simulink subsystem "ExcavatorLidarSensors"  (R2024a)
settings: Solver=VariableStepAuto  StartTime=0.0  StopTime=10.0  RelTol=1e-3
values from neighbouring files (symbols this model uses):
  lidarSampleTime = 0.1    [lidarSensorParameters.mat]
libraries: sim3dphyssensorlib x4
settings Model: Creator=ckammer  LastModifiedBy=ckammer

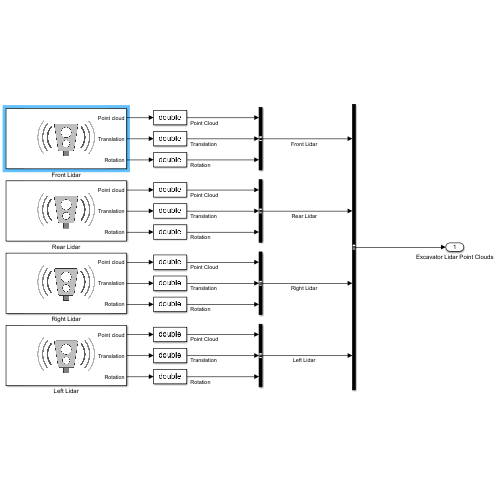
[thumbnail: Simulink's stored preview of the top-level diagram]
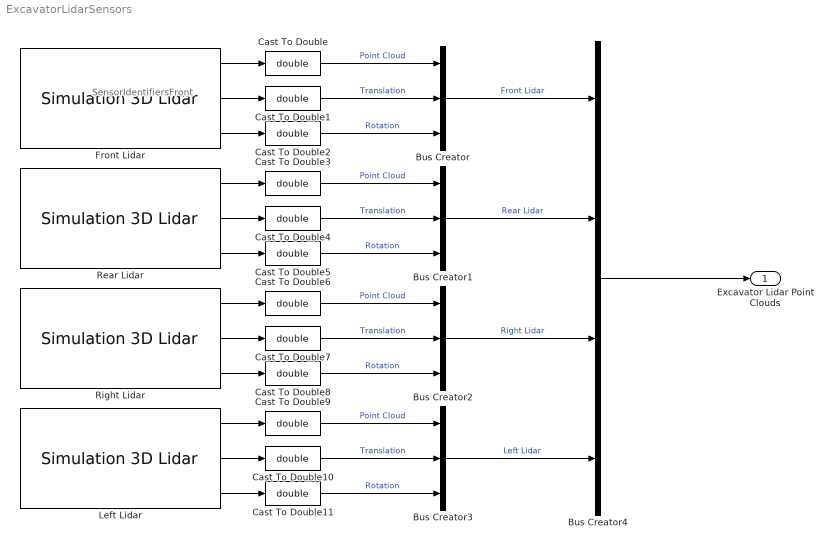
== system ExcavatorLidarSensors ==
  note: SensorIdentifiersFront
  Bus Creator{,1..3} (4 alike) : BusCreator  Inputs=3
  Bus Creator4 : BusCreator  Inputs=4
  Cast To Double{,1..11} (12 alike) : DataTypeConversion  OutDataTypeStr=double  SaturateOnIntegerOverflow=off  RndMeth=Floor
  Front Lidar : sim3dphyssensorlib/Simulation 3D Lidar  Priority=1  sensorTag=Sim3dSensorSensorIdentifiers.LidarSensorFront  sensorId=SensorIdentifiers.LidarSensorFront  sensorName=Sim3dSensorSensorIdentifiers.LidarSensorFront  vehTagList={'Scene Origin'}  vehTag=Scene Origin  mountLoc=Origin  offsetFlag=on  tmountOffset=lidarSensorOffsets.frontLidar.relativeTranslation  rmountOffset=lidarSensorOffsets.frontLidar.relativeRotation  DetectionRange=lidarPhysicalParams.DetectionRange  RangeResolution=0.002  VerticalFOV=lidarPhysicalParams.VerticalFieldOfView  VerticalResolution=1.25  HorizontalFOV=180  HorizontalResolution=0.16  DistanceOutportEnabled=off  ReflectivityOutportEnabled=off  SemanticOutportEnabled=off  TransformOutportEnabled=on  SampleTime=lidarSampleTime  mountPoint=[-1.4 3 0.7]  mountOrientation=[0 0 0]  aMode=5  ID=SensorIdentifiers.LidarSensorFront
      settings: LibrarySourceBlock=sl3dlib/Simulation 3D/Sensors/Simulation 3D Lidar
  Left Lidar : sim3dphyssensorlib/Simulation 3D Lidar  Priority=1  sensorTag=Sim3dSensorSensorIdentifiers.LidarSensorLeft  sensorId=SensorIdentifiers.LidarSensorLeft  sensorName=Sim3dSensorSensorIdentifiers.LidarSensorLeft  vehTagList={'Scene Origin'}  vehTag=Scene Origin  mountLoc=Origin  offsetFlag=on  tmountOffset=lidarSensorOffsets.leftLidar.relativeTranslation  rmountOffset=lidarSensorOffsets.leftLidar.relativeRotation  DetectionRange=lidarPhysicalParams.DetectionRange  RangeResolution=0.002  VerticalFOV=lidarPhysicalParams.VerticalFieldOfView  VerticalResolution=1.25  HorizontalFOV=180  HorizontalResolution=0.16  DistanceOutportEnabled=off  ReflectivityOutportEnabled=off  SemanticOutportEnabled=off  TransformOutportEnabled=on  SampleTime=lidarSampleTime  mountPoint=[1.5 -2.1 1.7]  mountOrientation=[0 0 -90]  aMode=5  ID=SensorIdentifiers.LidarSensorLeft
      settings: LibrarySourceBlock=sl3dlib/Simulation 3D/Sensors/Simulation 3D Lidar
  Rear Lidar : sim3dphyssensorlib/Simulation 3D Lidar  Priority=1  sensorTag=Sim3dSensorSensorIdentifiers.LidarSensorRear  sensorId=SensorIdentifiers.LidarSensorRear  sensorName=Sim3dSensorSensorIdentifiers.LidarSensorRear  vehTagList={'Scene Origin'}  vehTag=Scene Origin  mountLoc=Origin  offsetFlag=on  tmountOffset=lidarSensorOffsets.rearLidar.relativeTranslation  rmountOffset=lidarSensorOffsets.rearLidar.relativeRotation  DetectionRange=lidarPhysicalParams.DetectionRange  RangeResolution=0.002  VerticalFOV=lidarPhysicalParams.VerticalFieldOfView  VerticalResolution=1.25  HorizontalFOV=180  HorizontalResolution=0.16  DistanceOutportEnabled=off  ReflectivityOutportEnabled=off  SemanticOutportEnabled=off  TransformOutportEnabled=on  SampleTime=lidarSampleTime  mountPoint=[0.1 -4.2 1.7]  mountOrientation=[0 0 -180]  aMode=5  ID=SensorIdentifiers.LidarSensorRear
      settings: LibrarySourceBlock=sl3dlib/Simulation 3D/Sensors/Simulation 3D Lidar
  Right Lidar : sim3dphyssensorlib/Simulation 3D Lidar  Priority=1  sensorTag=Sim3dSensorSensorIdentifiers.LidarSensorRight  sensorId=SensorIdentifiers.LidarSensorRight  sensorName=Sim3dSensorSensorIdentifiers.LidarSensorRight  vehTagList={'Scene Origin'}  vehTag=Scene Origin  mountLoc=Origin  offsetFlag=on  tmountOffset=lidarSensorOffsets.rightLidar.relativeTranslation  rmountOffset=lidarSensorOffsets.rightLidar.relativeRotation  DetectionRange=lidarPhysicalParams.DetectionRange  RangeResolution=0.002  VerticalFOV=lidarPhysicalParams.VerticalFieldOfView  VerticalResolution=1.25  HorizontalFOV=180  HorizontalResolution=0.16  DistanceOutportEnabled=off  ReflectivityOutportEnabled=off  SemanticOutportEnabled=off  TransformOutportEnabled=on  SampleTime=lidarSampleTime  mountPoint=[-1.6 -2.1 1.7]  mountOrientation=[0 0 90]  aMode=5  ID=SensorIdentifiers.LidarSensorRight
      settings: LibrarySourceBlock=sl3dlib/Simulation 3D/Sensors/Simulation 3D Lidar
  Excavator Lidar Point Clouds : Outport
  wires:
  Front Lidar/1 -> Cast To Double/1
  Rear Lidar/1 -> Cast To Double3/1
  Right Lidar/1 -> Cast To Double6/1
  Left Lidar/1 -> Cast To Double9/1
  Bus Creator4/1 -> Excavator Lidar Point Clouds/1
  Front Lidar/2 -> Cast To Double1/1
  Front Lidar/3 -> Cast To Double2/1
  Rear Lidar/2 -> Cast To Double4/1
  Rear Lidar/3 -> Cast To Double5/1
  Right Lidar/2 -> Cast To Double7/1
  Right Lidar/3 -> Cast To Double8/1
  Left Lidar/2 -> Cast To Double10/1
  Left Lidar/3 -> Cast To Double11/1
  Bus Creator1/1 -> Bus Creator4/2  "Rear Lidar"
  Bus Creator2/1 -> Bus Creator4/3  "Right Lidar"
  Bus Creator3/1 -> Bus Creator4/4  "Left Lidar"
  Bus Creator/1 -> Bus Creator4/1  "Front Lidar"
  Cast To Double/1 -> Bus Creator/1  "Point Cloud"
  Cast To Double1/1 -> Bus Creator/2  "Translation"
  Cast To Double2/1 -> Bus Creator/3  "Rotation"
  Cast To Double3/1 -> Bus Creator1/1  "Point Cloud"
  Cast To Double4/1 -> Bus Creator1/2  "Translation"
  Cast To Double5/1 -> Bus Creator1/3  "Rotation"
  Cast To Double6/1 -> Bus Creator2/1  "Point Cloud"
  Cast To Double7/1 -> Bus Creator2/2  "Translation"
  Cast To Double8/1 -> Bus Creator2/3  "Rotation"
  Cast To Double9/1 -> Bus Creator3/1  "Point Cloud"
  Cast To Double10/1 -> Bus Creator3/2  "Translation"
  Cast To Double11/1 -> Bus Creator3/3  "Rotation"
